simulink model "testModel"  (R2022b)
settings: Solver=FixedStepAuto  StartTime=0.0  StopTime=inf  FixedStep=0.0005  RelTol=1e-3
libraries: BeamNG_interface x1
settings Model: Creator=matti  LastModifiedBy=matti

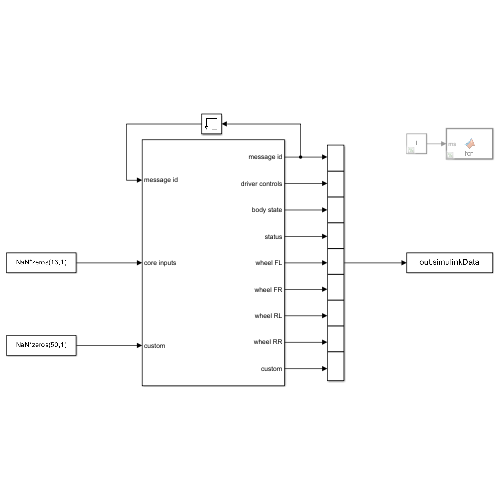
[thumbnail: Simulink's stored preview of the top-level diagram]
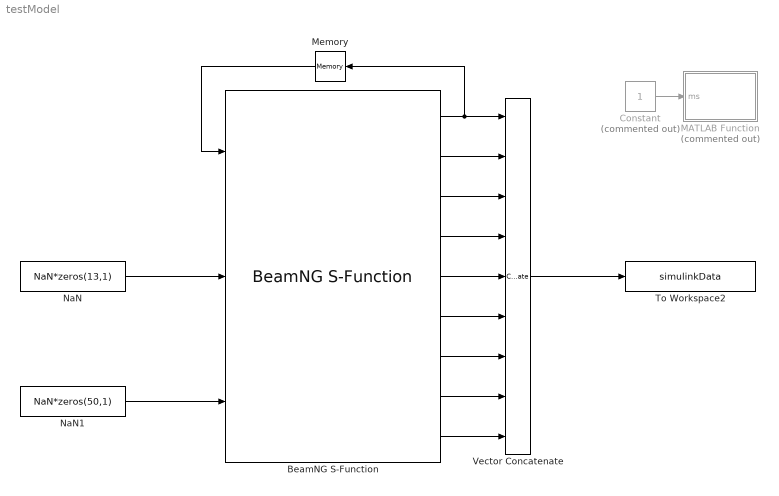
== system testModel ==
  BeamNG S-Function : BeamNG_interface/BeamNG S-Function  SFunctionModules=''
      settings: SourceProductName=BeamNG
  Constant : Constant  Commented=on
  MATLAB Function : MATLAB Function  Commented=on
  Memory : Memory
  NaN : Constant  Value=NaN*zeros(13,1)  OutDataTypeStr=Inherit: Inherit via back propagation
  NaN1 : Constant  Value=NaN*zeros(50,1)  OutDataTypeStr=Inherit: Inherit via back propagation
  To Workspace2 : ToWorkspace  VariableName=simulinkData  SaveFormat=Timeseries  SampleTime=-1
  Vector Concatenate : Concatenate  NumInputs=9
  wires:
  BeamNG S-Function/1 -> Vector Concatenate/1, Memory/1
  NaN/1 -> BeamNG S-Function/2
  BeamNG S-Function/9 -> Vector Concatenate/9
  BeamNG S-Function/8 -> Vector Concatenate/8
  BeamNG S-Function/7 -> Vector Concatenate/7
  BeamNG S-Function/6 -> Vector Concatenate/6
  BeamNG S-Function/5 -> Vector Concatenate/5
  BeamNG S-Function/4 -> Vector Concatenate/4
  BeamNG S-Function/2 -> Vector Concatenate/2
  BeamNG S-Function/3 -> Vector Concatenate/3
  Vector Concatenate/1 -> To Workspace2/1
  Memory/1 -> BeamNG S-Function/1
  NaN1/1 -> BeamNG S-Function/3
  Constant/1 -> MATLAB Function/1(ms)

== matlab function testModel/MATLAB Function ==
  data: ms input
function fcn(ms)

pause(ms / 1000);
